simulink model "GNC_physical_diagram"  (R2021b)
settings: Solver=VariableStepAuto  StartTime=0.0  StopTime=10.0  RelTol=1e-3
model workspace (MAT data in the model file):
  AV_Status_Signal : Simulink.Bus (value not decoded)
  Actuator_Signal : Simulink.Bus (value not decoded)
  Data_Stream : Simulink.Bus (value not decoded)
  Magnetororquer_Signal : Simulink.Bus (value not decoded)
  Mode_Trigger : Simulink.Bus (value not decoded)
  Reaction_Wheel_Signal : Simulink.Bus (value not decoded)
  Resources_Budget : Simulink.Bus (value not decoded)
  Sensor_Health : Simulink.Bus (value not decoded)
  Sensor_Signal : Simulink.Bus (value not decoded)
(part 2 of 2)

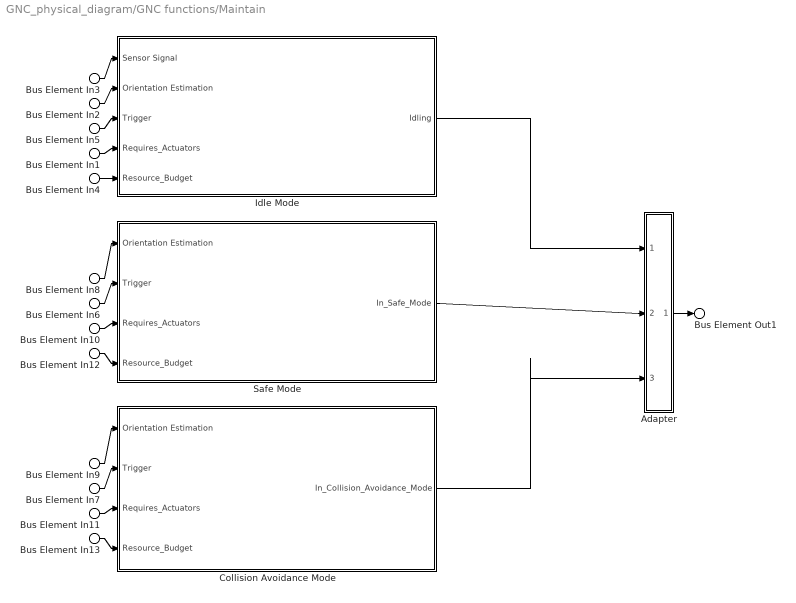
== system GNC_physical_diagram/GNC functions/Maintain ==
  Bus Element In3 : Inport  PortName=Sensor Signal
  Bus Element In2 : Inport  Port=2  PortName=Orientation Estimation
  Bus Element In8 : Inport  Port=2  PortName=Orientation Estimation
  Bus Element In9 : Inport  Port=2  PortName=Orientation Estimation
  Bus Element In6 : Inport  Port=3  PortName=Mode_Trigger  Element=Safe_Mode_Trigger
  Bus Element In7 : Inport  Port=3  PortName=Mode_Trigger  Element=Collision_Avoidance_Mode
  Bus Element In5 : Inport  Port=3  PortName=Mode_Trigger  Element=Idle_Mode_Trigger
  Bus Element In1 : Inport  Port=4  PortName=Requires_Actuators
  Bus Element In10 : Inport  Port=4  PortName=Requires_Actuators
  Bus Element In11 : Inport  Port=4  PortName=Requires_Actuators
  Bus Element In4 : Inport  Port=5  PortName=Resource_Budget
  Bus Element In12 : Inport  Port=5  PortName=Resource_Budget
  Bus Element In13 : Inport  Port=5  PortName=Resource_Budget
  Adapter : Subsystem
      settings: PortSchema="{\"entries\":[{\"content\":{\"margin\":10,\"minimumSpacing\":15,\"sides\":[{\"content\":{\"connectorIds\":[\"In1\",\"In2\",\"In3\"]},\"type\":\"ConnectorPlacement.EquallySpacedRectSide\",\"uuid\":\"04187947-a540-40f5-bdfb-67f982a6a3c9\"},{\"content\":{\"connectorIds\":[\"Out1\"],\"side\":\"RIGHT\"},\"type\":\"ConnectorPlacement.EquallySpacedRectSide\",\"uuid\":\"f31cf56a-b296-49ce-bb6c-3e31d54897fe\"},{\"content\":{\"connectorIds\":[],\"side\":\"TOP\"},\"type\":\"ConnectorPlacement.EquallySpacedRectSide\",\"uuid\":\"f63c8b68-6d1c-44a5-97b2-14525c5c4754\"}]},\"type\":\"ConnectorPlacement.EquallySpacedConnector\",\"uuid\":\"353cf843-0db6-4928-914d-fdc94187866a\"}],\"packageUris\":[\"http://schema.mathworks.com/mf0/Connector/R2020b\"],\"version\":\"1.0\"}"
  Collision Avoidance Mode : Subsystem
      settings: PortSchema="{\"entries\":[{\"content\":{\"headerSize\":26,\"margin\":15,\"minimumSpacing\":25,\"sides\":[{\"content\":{\"connectorIds\":[\"In1\",\"In2\",\"In3\",\"In4\"]},\"type\":\"ConnectorPlacement.EquallySpacedRectSide\",\"uuid\":\"04187947-a540-40f5-bdfb-67f982a6a3c9\"},{\"content\":{\"connectorIds\":[\"Out1\"],\"side\":\"RIGHT\"},\"type\":\"ConnectorPlacement.EquallySpacedRectSide\",\"uuid\":\"f31cf56a-b296-49ce-bb6c-3e31d54897fe\"},{\"content\":{\"connectorIds\":[],\"side\":\"TOP\"},\"type\":\"ConnectorPlacement.EquallySpacedRectSide\",\"uuid\":\"f63c8b68-6d1c-44a5-97b2-14525c5c4754\"}]},\"type\":\"ConnectorPlacement.EquallySpacedConnector\",\"uuid\":\"353cf843-0db6-4928-914d-fdc94187866a\"}],\"packageUris\":[\"http://schema.mathworks.com/mf0/Connector/R2020b\"],\"version\":\"1.0\"}"
  Idle Mode : Subsystem
      settings: PortSchema="{\"entries\":[{\"content\":{\"headerSize\":26,\"margin\":15,\"minimumSpacing\":25,\"sides\":[{\"content\":{\"connectorIds\":[\"In1\",\"In2\",\"In3\",\"In4\",\"In5\"]},\"type\":\"ConnectorPlacement.EquallySpacedRectSide\",\"uuid\":\"04187947-a540-40f5-bdfb-67f982a6a3c9\"},{\"content\":{\"connectorIds\":[\"Out1\"],\"side\":\"RIGHT\"},\"type\":\"ConnectorPlacement.EquallySpacedRectSide\",\"uuid\":\"f31cf56a-b296-49ce-bb6c-3e31d54897fe\"},{\"content\":{\"connectorIds\":[],\"side\":\"TOP\"},\"type\":\"ConnectorPlacement.EquallySpacedRectSide\",\"uuid\":\"f63c8b68-6d1c-44a5-97b2-14525c5c4754\"}]},\"type\":\"ConnectorPlacement.EquallySpacedConnector\",\"uuid\":\"353cf843-0db6-4928-914d-fdc94187866a\"}],\"packageUris\":[\"http://schema.mathworks.com/mf0/Connector/R2020b\"],\"version\":\"1.0\"}"
  Safe Mode : Subsystem
      settings: PortSchema="{\"entries\":[{\"content\":{\"headerSize\":26,\"margin\":15,\"minimumSpacing\":25,\"sides\":[{\"content\":{\"connectorIds\":[\"In1\",\"In2\",\"In3\",\"In4\"]},\"type\":\"ConnectorPlacement.EquallySpacedRectSide\",\"uuid\":\"04187947-a540-40f5-bdfb-67f982a6a3c9\"},{\"content\":{\"connectorIds\":[\"Out1\"],\"side\":\"RIGHT\"},\"type\":\"ConnectorPlacement.EquallySpacedRectSide\",\"uuid\":\"f31cf56a-b296-49ce-bb6c-3e31d54897fe\"},{\"content\":{\"connectorIds\":[],\"side\":\"TOP\"},\"type\":\"ConnectorPlacement.EquallySpacedRectSide\",\"uuid\":\"f63c8b68-6d1c-44a5-97b2-14525c5c4754\"}]},\"type\":\"ConnectorPlacement.EquallySpacedConnector\",\"uuid\":\"353cf843-0db6-4928-914d-fdc94187866a\"}],\"packageUris\":[\"http://schema.mathworks.com/mf0/Connector/R2020b\"],\"version\":\"1.0\"}"
  Bus Element Out1 : Outport  PortName=Maintaining
  wires:
  Bus Element In5/1 -> Idle Mode/3(Trigger)
  Bus Element In6/1 -> Safe Mode/2(Trigger)
  Bus Element In7/1 -> Collision Avoidance Mode/2(Trigger)
  Adapter/1(Maintaining) -> Bus Element Out1/1
  Idle Mode/1(Idling) -> Adapter/1(Idling)
  Safe Mode/1(In_Safe_Mode) -> Adapter/2(In_Safe_Mode)
  Collision Avoidance Mode/1(In_Collision_Avoidance_Mode) -> Adapter/3(In_Collision_Avoidance_Mode)
  Bus Element In2/1 -> Idle Mode/2(Orientation Estimation)
  Bus Element In8/1 -> Safe Mode/1(Orientation Estimation)
  Bus Element In3/1 -> Idle Mode/1(Sensor Signal)
  Bus Element In9/1 -> Collision Avoidance Mode/1(Orientation Estimation)
  Bus Element In1/1 -> Idle Mode/4(Requires_Actuators)
  Bus Element In10/1 -> Safe Mode/3(Requires_Actuators)
  Bus Element In11/1 -> Collision Avoidance Mode/3(Requires_Actuators)
  Bus Element In4/1 -> Idle Mode/5(Resource_Budget)
  Bus Element In12/1 -> Safe Mode/4(Resource_Budget)
  Bus Element In13/1 -> Collision Avoidance Mode/4(Resource_Budget)

== system GNC_physical_diagram/GNC functions/Recreation ==
  Bus Element In3 : Inport  PortName=Orientation Estimation
  Bus Element In4 : Inport  Port=2  PortName=Trigger
  Bus Element In1 : Inport  Port=3  PortName=Requires_Actuators
  Bus Element In2 : Inport  Port=4  PortName=Resource_Budget
  Bus Element Out1 : Outport  PortName=Recreation_Done

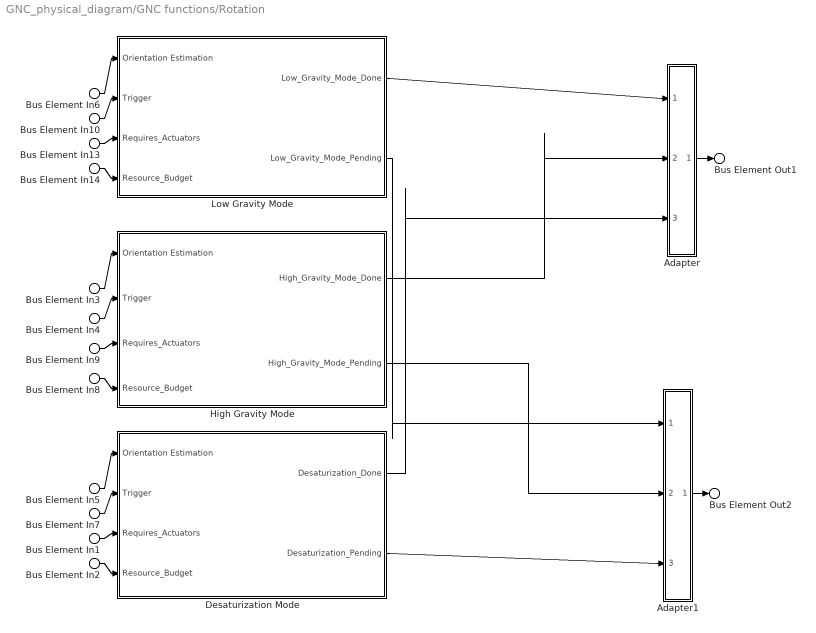
== system GNC_physical_diagram/GNC functions/Rotation ==
  Bus Element In3 : Inport  PortName=Orientation Estimation
  Bus Element In5 : Inport  PortName=Orientation Estimation
  Bus Element In6 : Inport  PortName=Orientation Estimation
  Bus Element In10 : Inport  Port=2  PortName=Mode_Trigger  Element=Low_Gravity_Mode_Trigger
  Bus Element In4 : Inport  Port=2  PortName=Mode_Trigger  Element=High_Gravity_Trigger
  Bus Element In7 : Inport  Port=2  PortName=Mode_Trigger  Element=Desaturization_Trigger
  Bus Element In1 : Inport  Port=3  PortName=Requires_Actuators
  Bus Element In9 : Inport  Port=3  PortName=Requires_Actuators
  Bus Element In13 : Inport  Port=3  PortName=Requires_Actuators
  Bus Element In2 : Inport  Port=4  PortName=Resource_Budget
  Bus Element In8 : Inport  Port=4  PortName=Resource_Budget
  Bus Element In14 : Inport  Port=4  PortName=Resource_Budget
  Adapter : Subsystem
      settings: PortSchema="{\"entries\":[{\"content\":{\"margin\":10,\"minimumSpacing\":15,\"sides\":[{\"content\":{\"connectorIds\":[\"In1\",\"In2\",\"In3\"]},\"type\":\"ConnectorPlacement.EquallySpacedRectSide\",\"uuid\":\"04187947-a540-40f5-bdfb-67f982a6a3c9\"},{\"content\":{\"connectorIds\":[\"Out1\"],\"side\":\"RIGHT\"},\"type\":\"ConnectorPlacement.EquallySpacedRectSide\",\"uuid\":\"f31cf56a-b296-49ce-bb6c-3e31d54897fe\"},{\"content\":{\"connectorIds\":[],\"side\":\"TOP\"},\"type\":\"ConnectorPlacement.EquallySpacedRectSide\",\"uuid\":\"f63c8b68-6d1c-44a5-97b2-14525c5c4754\"}]},\"type\":\"ConnectorPlacement.EquallySpacedConnector\",\"uuid\":\"353cf843-0db6-4928-914d-fdc94187866a\"}],\"packageUris\":[\"http://schema.mathworks.com/mf0/Connector/R2020b\"],\"version\":\"1.0\"}"
  Adapter1 : Subsystem
      settings: PortSchema="{\"entries\":[{\"content\":{\"margin\":10,\"minimumSpacing\":15,\"sides\":[{\"content\":{\"connectorIds\":[\"In1\",\"In2\",\"In3\"]},\"type\":\"ConnectorPlacement.EquallySpacedRectSide\",\"uuid\":\"04187947-a540-40f5-bdfb-67f982a6a3c9\"},{\"content\":{\"connectorIds\":[\"Out1\"],\"side\":\"RIGHT\"},\"type\":\"ConnectorPlacement.EquallySpacedRectSide\",\"uuid\":\"f31cf56a-b296-49ce-bb6c-3e31d54897fe\"},{\"content\":{\"connectorIds\":[],\"side\":\"TOP\"},\"type\":\"ConnectorPlacement.EquallySpacedRectSide\",\"uuid\":\"f63c8b68-6d1c-44a5-97b2-14525c5c4754\"}]},\"type\":\"ConnectorPlacement.EquallySpacedConnector\",\"uuid\":\"353cf843-0db6-4928-914d-fdc94187866a\"}],\"packageUris\":[\"http://schema.mathworks.com/mf0/Connector/R2020b\"],\"version\":\"1.0\"}"
  Desaturization Mode : Subsystem
      settings: PortSchema="{\"entries\":[{\"content\":{\"headerSize\":26,\"margin\":15,\"minimumSpacing\":25,\"sides\":[{\"content\":{\"connectorIds\":[\"In1\",\"In2\",\"In3\",\"In4\"]},\"type\":\"ConnectorPlacement.EquallySpacedRectSide\",\"uuid\":\"04187947-a540-40f5-bdfb-67f982a6a3c9\"},{\"content\":{\"connectorIds\":[\"Out1\",\"Out2\"],\"side\":\"RIGHT\"},\"type\":\"ConnectorPlacement.EquallySpacedRectSide\",\"uuid\":\"f31cf56a-b296-49ce-bb6c-3e31d54897fe\"},{\"content\":{\"connectorIds\":[],\"side\":\"TOP\"},\"type\":\"ConnectorPlacement.EquallySpacedRectSide\",\"uuid\":\"f63c8b68-6d1c-44a5-97b2-14525c5c4754\"}]},\"type\":\"ConnectorPlacement.EquallySpacedConnector\",\"uuid\":\"353cf843-0db6-4928-914d-fdc94187866a\"}],\"packageUris\":[\"http://schema.mathworks.com/mf0/Connector/R2020b\"],\"version\":\"1.0\"}"
  High Gravity Mode : Subsystem
      settings: PortSchema="{\"entries\":[{\"content\":{\"headerSize\":26,\"margin\":15,\"minimumSpacing\":25,\"sides\":[{\"content\":{\"connectorIds\":[\"In1\",\"In2\",\"In3\",\"In4\"]},\"type\":\"ConnectorPlacement.EquallySpacedRectSide\",\"uuid\":\"04187947-a540-40f5-bdfb-67f982a6a3c9\"},{\"content\":{\"connectorIds\":[\"Out1\",\"Out2\"],\"side\":\"RIGHT\"},\"type\":\"ConnectorPlacement.EquallySpacedRectSide\",\"uuid\":\"f31cf56a-b296-49ce-bb6c-3e31d54897fe\"},{\"content\":{\"connectorIds\":[],\"side\":\"TOP\"},\"type\":\"ConnectorPlacement.EquallySpacedRectSide\",\"uuid\":\"f63c8b68-6d1c-44a5-97b2-14525c5c4754\"}]},\"type\":\"ConnectorPlacement.EquallySpacedConnector\",\"uuid\":\"353cf843-0db6-4928-914d-fdc94187866a\"}],\"packageUris\":[\"http://schema.mathworks.com/mf0/Connector/R2020b\"],\"version\":\"1.0\"}"
  Low Gravity Mode : Subsystem
      settings: PortSchema="{\"entries\":[{\"content\":{\"headerSize\":26,\"margin\":15,\"minimumSpacing\":25,\"sides\":[{\"content\":{\"connectorIds\":[\"In1\",\"In4\",\"In2\",\"In3\"]},\"type\":\"ConnectorPlacement.EquallySpacedRectSide\",\"uuid\":\"04187947-a540-40f5-bdfb-67f982a6a3c9\"},{\"content\":{\"connectorIds\":[\"Out1\",\"Out2\"],\"side\":\"RIGHT\"},\"type\":\"ConnectorPlacement.EquallySpacedRectSide\",\"uuid\":\"f31cf56a-b296-49ce-bb6c-3e31d54897fe\"},{\"content\":{\"connectorIds\":[],\"side\":\"TOP\"},\"type\":\"ConnectorPlacement.EquallySpacedRectSide\",\"uuid\":\"f63c8b68-6d1c-44a5-97b2-14525c5c4754\"}]},\"type\":\"ConnectorPlacement.EquallySpacedConnector\",\"uuid\":\"353cf843-0db6-4928-914d-fdc94187866a\"}],\"packageUris\":[\"http://schema.mathworks.com/mf0/Connector/R2020b\"],\"version\":\"1.0\"}"
  Bus Element Out1 : Outport  PortName=Rotation_Done
  Bus Element Out2 : Outport  Port=2  PortName=Is_Rotating
  wires:
  Bus Element In2/1 -> Desaturization Mode/4(Resource_Budget)
  Bus Element In8/1 -> High Gravity Mode/4(Resource_Budget)
  Bus Element In1/1 -> Desaturization Mode/3(Requires_Actuators)
  Bus Element In9/1 -> High Gravity Mode/3(Requires_Actuators)
  Bus Element In3/1 -> High Gravity Mode/1(Orientation Estimation)
  Bus Element In5/1 -> Desaturization Mode/1(Orientation Estimation)
  Bus Element In6/1 -> Low Gravity Mode/1(Orientation Estimation)
  Bus Element In13/1 -> Low Gravity Mode/2(Requires_Actuators)
  Bus Element In14/1 -> Low Gravity Mode/3(Resource_Budget)
  Adapter/1(Rotation_Done) -> Bus Element Out1/1
  Adapter1/1(Is_Rotating) -> Bus Element Out2/1
  Low Gravity Mode/1(Low_Gravity_Mode_Done) -> Adapter/1(Low_Gravity_Mode_Done)
  High Gravity Mode/1(High_Gravity_Mode_Done) -> Adapter/2(High_Gravity_Mode_Done)
  Desaturization Mode/1(Desaturization_Done) -> Adapter/3(Desaturization_Done)
  High Gravity Mode/2(High_Gravity_Mode_Pending) -> Adapter1/2(High_Gravity_Mode_Pending)
  Low Gravity Mode/2(Low_Gravity_Mode_Pending) -> Adapter1/1(Low_Gravity_Mode_Pending)
  Desaturization Mode/2(Desaturization_Pending) -> Adapter1/3(Desaturization_Pending)
  Bus Element In10/1 -> Low Gravity Mode/4(Trigger)
  Bus Element In4/1 -> High Gravity Mode/2(Trigger)
  Bus Element In7/1 -> Desaturization Mode/2(Trigger)

== system GNC_physical_diagram/GNC functions/Testing ==
  Bus Element In1 : Inport  PortName=Trigger
  Bus Element In3 : Inport  Port=2  PortName=Requires_Actuators
  Bus Element In2 : Inport  Port=3  PortName=Resource_Budget
  Bus Element Out1 : Outport  PortName=Testing_Done

== system GNC_physical_diagram/Orientation Estimation/Sensor Elimination ==
  Bus Element In1 : Inport  PortName=Sensor Signal
  Bus Element Out2 : Outport  PortName=Sensor_Health

== system GNC_physical_diagram/Sensors/Adapter ==
  In Bus Element : Inport  PortName=Sun_Sensor_Signal
  Bus Element In2 : Inport  Port=2  PortName=Magnetometer_Signal
  Bus Element In3 : Inport  Port=3  PortName=IMU_signal
  Bus Element In4 : Inport  Port=4  PortName=GPS_Signal
  Out Bus Element : Outport  PortName=Sensor Signal
  wires:
  In Bus Element/1 -> Out Bus Element/1

== system GNC_physical_diagram/Sensors/GPS ==
  Bus Element In1 : Inport  PortName=Disturbances
  Bus Element In2 : Inport  Port=2  PortName=Resource_Budget
  Bus Element Out1 : Outport  PortName=GPS_Signal

== system GNC_physical_diagram/Sensors/IMUs ==
  Bus Element In1 : Inport  PortName=Disturbances
  Bus Element In2 : Inport  Port=2  PortName=Resource_Budget
  Bus Element Out1 : Outport  PortName=IMU_signal

== system GNC_physical_diagram/Sensors/Magnetometers ==
  Bus Element In1 : Inport  PortName=Disturbances
  Bus Element In2 : Inport  Port=2  PortName=Resource_Budget
  Bus Element Out1 : Outport  PortName=Magnetometer_Signal

== system GNC_physical_diagram/Sensors/Sun Sensors ==
  Bus Element In1 : Inport  PortName=Disturbances
  Bus Element In2 : Inport  Port=2  PortName=Resource_Budget
  Bus Element Out1 : Outport  PortName=Sun_Sensor_Signal

== system GNC_physical_diagram/Actuators/Magnetorquers/Adapter ==
  In Bus Element : Inport  PortName=Heat 1
  Bus Element In2 : Inport  Port=2  PortName=Heat 2
  Bus Element In3 : Inport  Port=3  PortName=Heat 3
  Bus Element In4 : Inport  Port=4  PortName=Heat 4
  Out Bus Element : Outport  PortName=Coil_Heat
  wires:
  In Bus Element/1 -> Out Bus Element/1

== system GNC_physical_diagram/Actuators/Magnetorquers/Adapter1 ==
  In Bus Element : Inport  PortName=Torque 1
  Bus Element In2 : Inport  Port=2  PortName=Torque 2
  Bus Element In3 : Inport  Port=3  PortName=Torque 3
  Bus Element In4 : Inport  Port=4  PortName=Torque 4
  Out Bus Element : Outport  PortName=Magnetic_Torque
  wires:
  In Bus Element/1 -> Out Bus Element/1

== system GNC_physical_diagram/Actuators/Magnetorquers/Magnetotorquer 1 ==
  Bus Element In1 : Inport  PortName=Power
  Bus Element In2 : Inport  Port=2  PortName=Signal
  Bus Element Out1 : Outport  PortName=Heat 1
  Bus Element Out2 : Outport  Port=2  PortName=Torque 1

== system GNC_physical_diagram/Actuators/Magnetorquers/Magnetotorquer 2 ==
  Bus Element In1 : Inport  PortName=Power
  Bus Element In2 : Inport  Port=2  PortName=Signal
  Bus Element Out1 : Outport  PortName=Heat 2
  Bus Element Out2 : Outport  Port=2  PortName=Torque 2

== system GNC_physical_diagram/Actuators/Magnetorquers/Magnetotorquer 3 ==
  Bus Element In1 : Inport  PortName=Power
  Bus Element In2 : Inport  Port=2  PortName=Signal
  Bus Element Out1 : Outport  PortName=Heat 3
  Bus Element Out2 : Outport  Port=2  PortName=Torque 3

== system GNC_physical_diagram/Actuators/Magnetorquers/Magnetotorquer 4 ==
  Bus Element In1 : Inport  PortName=Power
  Bus Element In2 : Inport  Port=2  PortName=Signal
  Bus Element Out1 : Outport  PortName=Heat 4
  Bus Element Out2 : Outport  Port=2  PortName=Torque 4

== system GNC_physical_diagram/Actuators/Reaction Wheels/Adapter ==
  In Bus Element : Inport  PortName=Heat 1
  Bus Element In2 : Inport  Port=2  PortName=Heat 2
  Bus Element In3 : Inport  Port=3  PortName=Heat 3
  Bus Element In4 : Inport  Port=4  PortName=Heat 4
  Out Bus Element : Outport  PortName=Motor_Heat
  wires:
  In Bus Element/1 -> Out Bus Element/1

== system GNC_physical_diagram/Actuators/Reaction Wheels/Adapter1 ==
  In Bus Element : Inport  PortName=Torque 1
  Bus Element In2 : Inport  Port=2  PortName=Torque 2
  Bus Element In3 : Inport  Port=3  PortName=Torque 4
  Bus Element In4 : Inport  Port=4  PortName=InBus
  Out Bus Element : Outport  PortName=Reaction_Torque
  wires:
  In Bus Element/1 -> Out Bus Element/1

== system GNC_physical_diagram/Actuators/Reaction Wheels/Adapter2 ==
  In Bus Element : Inport  PortName=Signal 1
  Bus Element In2 : Inport  Port=2  PortName=Signal 2
  Bus Element In3 : Inport  Port=3  PortName=Signal 3
  Bus Element In4 : Inport  Port=4  PortName=Signal 4
  Out Bus Element : Outport  PortName=Encoder Signal
  wires:
  In Bus Element/1 -> Out Bus Element/1

== system GNC_physical_diagram/Actuators/Reaction Wheels/Reaction Wheel 1 ==
  Bus Element In1 : Inport  PortName=Power
  Bus Element In2 : Inport  Port=2  PortName=Signal
  Bus Element Out1 : Outport  PortName=Heat 1
  Bus Element Out2 : Outport  Port=2  PortName=Torque 1
  Bus Element Out3 : Outport  Port=3  PortName=Signal 1

== system GNC_physical_diagram/Actuators/Reaction Wheels/Reaction Wheel 2 ==
  Bus Element In1 : Inport  PortName=Power
  Bus Element In2 : Inport  Port=2  PortName=Signal
  Bus Element Out1 : Outport  PortName=Heat 2
  Bus Element Out2 : Outport  Port=2  PortName=Torque 2
  Bus Element Out3 : Outport  Port=3  PortName=Signal 2

== system GNC_physical_diagram/Actuators/Reaction Wheels/Reaction Wheel 3 ==
  Bus Element In1 : Inport  PortName=Power
  Bus Element In2 : Inport  Port=2  PortName=Signal
  Bus Element Out1 : Outport  PortName=Heat 3
  Bus Element Out2 : Outport  Port=2  PortName=Torque 3
  Bus Element Out3 : Outport  Port=3  PortName=Signal 3

== system GNC_physical_diagram/Actuators/Reaction Wheels/Reaction Wheel 4 ==
  Bus Element In1 : Inport  PortName=Power
  Bus Element In2 : Inport  Port=2  PortName=Signal
  Bus Element Out1 : Outport  PortName=Heat 4
  Bus Element Out2 : Outport  Port=2  PortName=Torque 4
  Bus Element Out3 : Outport  Port=3  PortName=Signal 4

== system GNC_physical_diagram/Avionics Hardware/Ground Station/Trajectory Estimation ==
  Bus Element In2 : Inport  PortName=Orientation Estimation
  Bus Element In1 : Inport  Port=2  PortName=Loggable Data
  Bus Element Out1 : Outport  PortName=Trajectory

== system GNC_physical_diagram/GNC functions/Maintain/Adapter ==
  In Bus Element : Inport  PortName=Idling
  Bus Element In2 : Inport  Port=2  PortName=In_Safe_Mode
  Bus Element In3 : Inport  Port=3  PortName=In_Collision_Avoidance_Mode
  Out Bus Element : Outport  PortName=Maintaining
  wires:
  In Bus Element/1 -> Out Bus Element/1

== system GNC_physical_diagram/GNC functions/Maintain/Collision Avoidance Mode ==
  Bus Element In2 : Inport  PortName=Orientation Estimation
  Bus Element In1 : Inport  Port=2  PortName=Trigger
  Bus Element In3 : Inport  Port=3  PortName=Requires_Actuators
  Bus Element In4 : Inport  Port=4  PortName=Resource_Budget
  Bus Element Out1 : Outport  PortName=In_Collision_Avoidance_Mode

== system GNC_physical_diagram/GNC functions/Maintain/Idle Mode ==
  Bus Element In3 : Inport  PortName=Sensor Signal
  Bus Element In2 : Inport  Port=2  PortName=Orientation Estimation
  Bus Element In1 : Inport  Port=3  PortName=Trigger
  Bus Element In4 : Inport  Port=4  PortName=Requires_Actuators
  Bus Element In5 : Inport  Port=5  PortName=Resource_Budget
  Bus Element Out1 : Outport  PortName=Idling

== system GNC_physical_diagram/GNC functions/Maintain/Safe Mode ==
  Bus Element In2 : Inport  PortName=Orientation Estimation
  Bus Element In1 : Inport  Port=2  PortName=Trigger
  Bus Element In3 : Inport  Port=3  PortName=Requires_Actuators
  Bus Element In4 : Inport  Port=4  PortName=Resource_Budget
  Bus Element Out1 : Outport  PortName=In_Safe_Mode

== system GNC_physical_diagram/GNC functions/Rotation/Adapter ==
  In Bus Element : Inport  PortName=Low_Gravity_Mode_Done
  Bus Element In2 : Inport  Port=2  PortName=High_Gravity_Mode_Done
  Bus Element In3 : Inport  Port=3  PortName=Desaturization_Done
  Out Bus Element : Outport  PortName=Rotation_Done
  wires:
  In Bus Element/1 -> Out Bus Element/1

== system GNC_physical_diagram/GNC functions/Rotation/Adapter1 ==
  Bus Element In1 : Inport  PortName=Low_Gravity_Mode_Pending
  Bus Element In2 : Inport  Port=2  PortName=High_Gravity_Mode_Pending
  Bus Element In3 : Inport  Port=3  PortName=Desaturization_Pending
  Out Bus Element : Outport  PortName=Is_Rotating

== system GNC_physical_diagram/GNC functions/Rotation/Desaturization Mode ==
  Bus Element In2 : Inport  PortName=Orientation Estimation
  Bus Element In4 : Inport  Port=2  PortName=Trigger
  Bus Element In3 : Inport  Port=3  PortName=Requires_Actuators
  Bus Element In1 : Inport  Port=4  PortName=Resource_Budget
  Bus Element Out1 : Outport  PortName=Desaturization_Done
  Bus Element Out2 : Outport  Port=2  PortName=Desaturization_Pending

== system GNC_physical_diagram/GNC functions/Rotation/High Gravity Mode ==
  Bus Element In1 : Inport  PortName=Orientation Estimation
  Bus Element In4 : Inport  Port=2  PortName=Trigger
  Bus Element In3 : Inport  Port=3  PortName=Requires_Actuators
  Bus Element In2 : Inport  Port=4  PortName=Resource_Budget
  Bus Element Out1 : Outport  PortName=High_Gravity_Mode_Done
  Bus Element Out2 : Outport  Port=2  PortName=High_Gravity_Mode_Pending

== system GNC_physical_diagram/GNC functions/Rotation/Low Gravity Mode ==
  Bus Element In1 : Inport  PortName=Orientation Estimation
  Bus Element In3 : Inport  Port=2  PortName=Requires_Actuators
  Bus Element In4 : Inport  Port=3  PortName=Resource_Budget
  Bus Element In5 : Inport  Port=4  PortName=Trigger
  Bus Element Out1 : Outport  PortName=Low_Gravity_Mode_Done
  Bus Element Out2 : Outport  Port=2  PortName=Low_Gravity_Mode_Pending
